simulink model "car_PID_sphi"  (R2019a)
settings: Solver=VariableStepAuto  StartTime=0.0  StopTime=10  RelTol=1e-3
values from neighbouring files (symbols this model uses):
  A = [-0.231185976061678;-0.498866089249557;5.84393669821388;3.73021803318506;9.90763303129933]    [rlocus.m]
  B = [4.16554325826943;-0.893946443952200;43.7489661560407;792.115696320530;120.101219035737]    [rlocus.m]
undefined symbols (not defined in the file or in its folder): DiscIntNeverNeededParam
libraries: simulink x1
settings Model: Creator=ray  LastModifiedBy=USER
settings DebuggingCC: AlgebraicLoopMsg=none

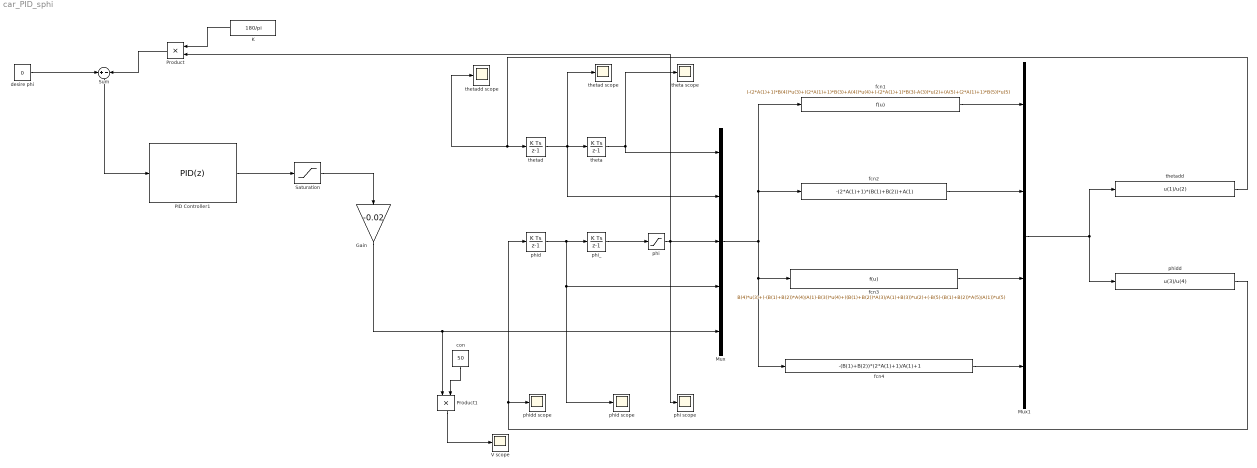
== system car_PID_sphi ==
  Gain : Gain  Gain=-0.02
  "K " : Constant  Value=180/pi  SampleTime=0.01
  Mux : Mux  Inputs=5
  Mux1 : Mux
  PID Controller1 : simulink/Continuous/PID Controller  Controller=PID  Form=Parallel  TimeDomain=Discrete-time  SampleTime=0.001  IntegratorMethod=Forward Euler  FilterMethod=Forward Euler  ControllerParametersSource=internal  P=10  I=100  D=0.01  UseFilter=on  N=100  TunerSelectOption=Transfer Function Based (PID Tuner App)  InitialConditionSource=internal  InitialConditionForIntegrator=0  InitialConditionForFilter=0  DifferentiatorICPrevScaledInput=0  ExternalReset=none  TrackingMode=off  Kt=1  LimitOutput=off  UpperSaturationLimit=inf  LowerSaturationLimit=-inf  LinearizeAsGain=on  AntiWindupMode=none  Kb=1  POutMin=[]  POutMax=[]  IOutMin=[]  IOutMax=[]  DOutMin=[]  DOutMax=[]  NOutMin=[]  NOutMax=[]  SumOutMin=[]  SumOutMax=[]  SaturationOutMin=[]  SaturationOutMax=[]  PParamMin=[]  PParamMax=[]  IParamMin=[]  IParamMax=[]  DParamMin=[]  DParamMax=[]  NParamMin=[]  NParamMax=[]  KbParamMin=[]  KbParamMax=[]  KtParamMin=[]  KtParamMax=[]  KbOutMin=[]  KbOutMax=[]  KtOutMin=[]  KtOutMax=[]  IntegratorOutMin=[]  IntegratorOutMax=[]  FilterOutMin=[]  FilterOutMax=[]  SumI1OutMin=[]  SumI1OutMax=[]  SumI2OutMin=[]  SumI2OutMax=[]  SumI3OutMin=[]  SumI3OutMax=[]  SumI4OutMin=[]  SumI4OutMax=[]  SumDOutMin=[]  SumDOutMax=[]  DifferentiatorOutMin=[]  DifferentiatorOutMax=[]  FilterDiffOutCoefMin=[]  FilterDiffOutCoefMax=[]  ReciprocalOutMin=[]  ReciprocalOutMax=[]  SumDenOutMin=[]  SumDenOutMax=[]  SumNumOutMin=[]  SumNumOutMax=[]  DivideOutMin=[]  DivideOutMax=[]  IntegratorContinuousStateAttributes=''  IntegratorStateMustResolveToSignalObject=off  IntegratorRTWStateStorageClass=Auto  FilterContinuousStateAttributes=''  FilterStateMustResolveToSignalObject=off  FilterRTWStateStorageClass=Auto  ParallelPVariant=InternalParameters  IdealPVariant=Disabled  IVariant=InternalParameters  DVariant=InternalParameters  IntegratorVariant=Discrete  SatVariant=Disabled  AWVariant=Passthrough  PCopyVariant=Disabled  TRVariant=Disabled  FdbkBlocksVariant=Forward  IdealPFdbkVariant=Disabled  SatFdbkVariant=Disabled  DerivativeFilterVariant=ForwardEulerFilter  NVariant=InternalParameters  NCopyVariant=Disabled  FilterICVariant=InternalICsFilter  IntegratorICVariant=InternalICs  ExternalResetVariant=Disabled  TRSumVariant=Passthrough  SumFdbkVariant=Disabled  SumVariant=Sum_PID
  Product : Product
  Product1 : Product
  Saturation : Saturate  UpperLimit=100  LowerLimit=-100
  Sum : Sum  Inputs=+-
  "V scope " : Scope
  "con " : Constant  Value=50  SampleTime=0.01
  "desire phi " : Constant  Value=0  SampleTime=0.001
  fcn1 : Fcn  Expr=(-(2*A(1)+1)*B(4))*u(3)+((2*A(1)+1)*B(3)+A(4))*u(4)+(-(2*A(1)+1)*B(3)-A(3))*u(2)+(A(5)+(2*A(1)+1)*B(5))*u(5)
  fcn2 : Fcn  Expr=-(2*A(1)+1)*(B(1)+B(2))+A(1)
  fcn3 : Fcn  Expr=B(4)*u(3)+(-(B(1)+B(2))*A(4)/A(1)-B(3))*u(4)+((B(1)+B(2))*A(3)/A(1)+B(3))*u(2)+(-B(5)-(B(1)+B(2))*A(5)/A(1))*u(5)
  fcn4 : Fcn  Expr=-(B(1)+B(2))*(2*A(1)+1)/A(1)+1
  phi : Saturate  UpperLimit=1.6  LowerLimit=-1.6
  "phi scope " : Scope
  phi_ : DiscreteIntegrator  InitialCondition=-0.01  SampleTime=0.001  ICPrevOutput=DiscIntNeverNeededParam  ICPrevScaledInput=DiscIntNeverNeededParam
  phid : DiscreteIntegrator  SampleTime=0.001  ICPrevOutput=DiscIntNeverNeededParam  ICPrevScaledInput=DiscIntNeverNeededParam
  "phid scope " : Scope
  phidd : Fcn  Expr=u(3)/u(4)
  "phidd scope " : Scope
  theta : DiscreteIntegrator  SampleTime=0.001  ICPrevOutput=DiscIntNeverNeededParam  ICPrevScaledInput=DiscIntNeverNeededParam
  theta scope : Scope
  thetad : DiscreteIntegrator  SampleTime=0.001  ICPrevOutput=DiscIntNeverNeededParam  ICPrevScaledInput=DiscIntNeverNeededParam
  "thetad scope " : Scope
  thetadd : Fcn  Expr=u(1)/u(2)
  "thetadd scope " : Scope
  wires:
  phid/1 -> Mux/4, "phid scope "/1, phi_/1
  phi_/1 -> phi/1
  phi/1 -> Product/2, Mux/3, "phi scope "/1
  Gain/1 -> Mux/5, Product1/1
  fcn4/1 -> Mux1/4
  fcn3/1 -> Mux1/3
  fcn2/1 -> Mux1/2
  fcn1/1 -> Mux1/1
  theta/1 -> theta scope/1, Mux/1
  Mux1/1 -> phidd/1, thetadd/1
  Mux/1 -> fcn2/1, fcn1/1, fcn4/1, fcn3/1
  thetad/1 -> "thetad scope "/1, Mux/2, theta/1
  thetadd/1 -> "thetadd scope "/1, thetad/1
  phidd/1 -> phid/1, "phidd scope "/1
  PID Controller1/1 -> Saturation/1
  Saturation/1 -> Gain/1
  "desire phi "/1 -> Sum/1
  Sum/1 -> PID Controller1/1
  "K "/1 -> Product/1
  Product/1 -> Sum/2
  Product1/1 -> "V scope "/1
  "con "/1 -> Product1/2
